simulink model "plant_ode_tmp"  (R2023b)
settings: Solver=VariableStepAuto  StartTime=0.0  StopTime=10.0  RelTol=1e-3
values from neighbouring files (symbols this model uses):
  param = plant_param()    [plot_bode.m]    (also in plot_impulse.m; plot_initial.m)
  x0 = [0;0;50e3;50e3]    [plot_initial.m]
libraries: simulink x4
settings Model: Creator=block  LastModifiedBy=MPC5

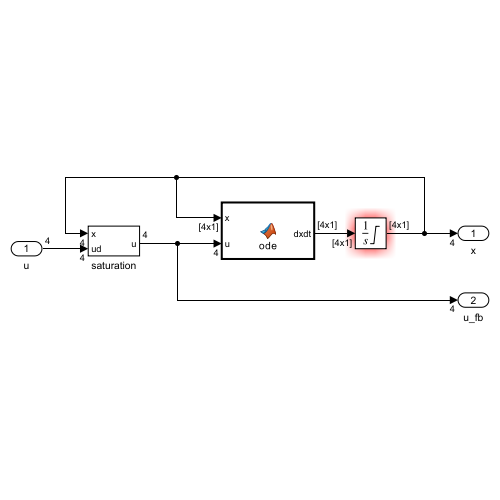
[thumbnail: Simulink's stored preview of the top-level diagram]
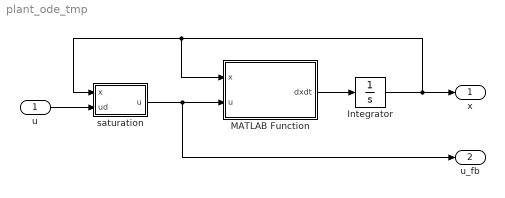
== system plant_ode_tmp ==
  u : Inport  PortDimensions=param.udim
  Integrator : Integrator  InitialCondition=x0  LimitOutput=on  UpperSaturationLimit=[param.L/2;inf;inf;inf]  LowerSaturationLimit=[-param.L/2;-inf;-inf;-inf]
  MATLAB Function : MATLAB Function  TreatAsAtomicUnit=on
  saturation : Subsystem
  x : Outport  PortDimensions=param.xdim
  u_fb : Outport  Port=2  PortDimensions=param.udim
  wires:
  MATLAB Function/1(dxdt) -> Integrator/1
  Integrator/1 -> x/1, MATLAB Function/1(x), saturation/1(x)
  saturation/1(u) -> u_fb/1, MATLAB Function/2(u)
  u/1 -> saturation/2(ud)

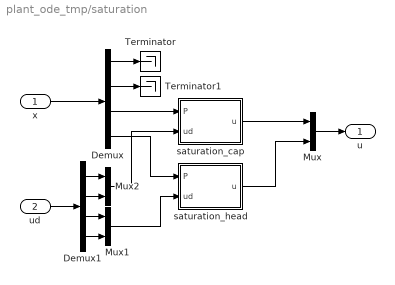
== system plant_ode_tmp/saturation ==
  x : Inport  PortDimensions=param.xdim
  ud : Inport  Port=2  PortDimensions=param.udim
  Demux : Demux
  Demux1 : Demux
  Mux : Mux  Inputs=2
  Mux1 : Mux  Inputs=2
  Mux2 : Mux  Inputs=2
  Terminator : Terminator
  Terminator1 : Terminator
  saturation_cap : Subsystem
  saturation_head : Subsystem
  u : Outport
  wires:
  x/1 -> Demux/1
  Demux/3 -> saturation_cap/1(P)
  Demux/4 -> saturation_head/1(P)
  Demux/1 -> Terminator/1
  Demux/2 -> Terminator1/1
  saturation_cap/1(u) -> Mux/1
  saturation_head/1(u) -> Mux/2
  Mux/1 -> u/1
  ud/1 -> Demux1/1
  Demux1/4 -> Mux1/2
  Demux1/3 -> Mux1/1
  Demux1/1 -> Mux2/1
  Demux1/2 -> Mux2/2
  Mux2/1 -> saturation_cap/2(ud)
  Mux1/1 -> saturation_head/2(ud)

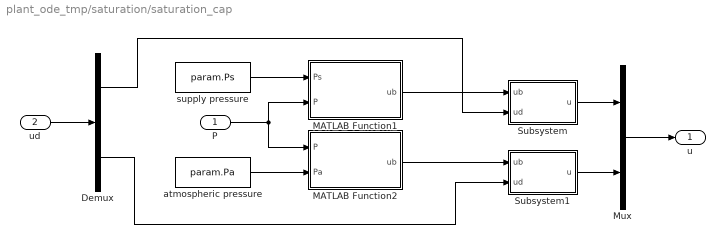
== system plant_ode_tmp/saturation/saturation_cap ==
  P : Inport
  ud : Inport  Port=2
  Demux : Demux  Outputs=2
  MATLAB Function1 : MATLAB Function  TreatAsAtomicUnit=on
  MATLAB Function2 : MATLAB Function  TreatAsAtomicUnit=on
  Mux : Mux  Inputs=2
  Subsystem : Subsystem
  Subsystem1 : Subsystem
  atmospheric pressure : Constant  Value=param.Pa
  supply pressure : Constant  Value=param.Ps
  u : Outport
  wires:
  ud/1 -> Demux/1
  Mux/1 -> u/1
  supply pressure/1 -> MATLAB Function1/1(Ps)
  P/1 -> MATLAB Function1/2(P), MATLAB Function2/1(P)
  atmospheric pressure/1 -> MATLAB Function2/2(Pa)
  MATLAB Function1/1(ub) -> Subsystem/1(ub)
  MATLAB Function2/1(ub) -> Subsystem1/1(ub)
  Demux/1 -> Subsystem/2(ud)
  Demux/2 -> Subsystem1/2(ud)
  Subsystem/1(u) -> Mux/1
  Subsystem1/1(u) -> Mux/2

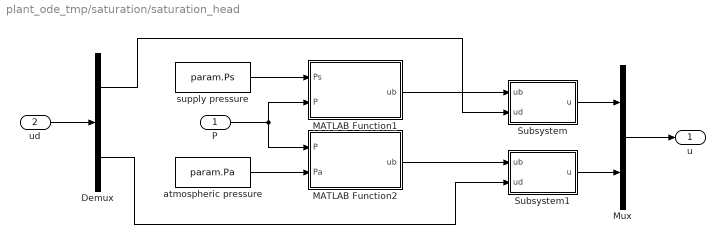
== system plant_ode_tmp/saturation/saturation_head ==
  P : Inport
  ud : Inport  Port=2
  Demux : Demux  Outputs=2
  MATLAB Function1 : MATLAB Function  TreatAsAtomicUnit=on
  MATLAB Function2 : MATLAB Function  TreatAsAtomicUnit=on
  Mux : Mux  Inputs=2
  Subsystem : Subsystem
  Subsystem1 : Subsystem
  atmospheric pressure : Constant  Value=param.Pa
  supply pressure : Constant  Value=param.Ps
  u : Outport
  wires:
  ud/1 -> Demux/1
  Mux/1 -> u/1
  supply pressure/1 -> MATLAB Function1/1(Ps)
  P/1 -> MATLAB Function1/2(P), MATLAB Function2/1(P)
  atmospheric pressure/1 -> MATLAB Function2/2(Pa)
  MATLAB Function1/1(ub) -> Subsystem/1(ub)
  MATLAB Function2/1(ub) -> Subsystem1/1(ub)
  Demux/1 -> Subsystem/2(ud)
  Demux/2 -> Subsystem1/2(ud)
  Subsystem/1(u) -> Mux/1
  Subsystem1/1(u) -> Mux/2

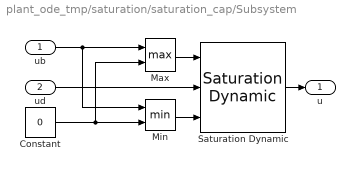
== system plant_ode_tmp/saturation/saturation_cap/Subsystem ==
  ub : Inport
  ud : Inport  Port=2
  Constant : Constant  Value=0
  Max : MinMax  Function=max  Inputs=2
  Min : MinMax  Inputs=2
  Saturation Dynamic : simulink/Discontinuities/Saturation Dynamic  OutMin=[]  OutMax=[]  OutDataTypeStr=Inherit: Same as second input  OutDataType=fixdt(1, 16)  OutScaling=2^-10  DoSatur=off
  u : Outport
  wires:
  Min/1 -> Saturation Dynamic/3
  ud/1 -> Saturation Dynamic/2
  Constant/1 -> Max/2, Min/2
  Max/1 -> Saturation Dynamic/1
  Saturation Dynamic/1 -> u/1
  ub/1 -> Min/1, Max/1

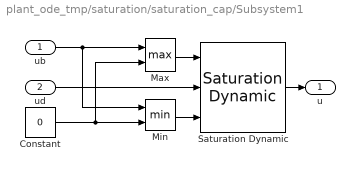
== system plant_ode_tmp/saturation/saturation_cap/Subsystem1 ==
  ub : Inport
  ud : Inport  Port=2
  Constant : Constant  Value=0
  Max : MinMax  Function=max  Inputs=2
  Min : MinMax  Inputs=2
  Saturation Dynamic : simulink/Discontinuities/Saturation Dynamic  OutMin=[]  OutMax=[]  OutDataTypeStr=Inherit: Same as second input  OutDataType=fixdt(1, 16)  OutScaling=2^-10  DoSatur=off
  u : Outport
  wires:
  ub/1 -> Max/1, Min/1
  Saturation Dynamic/1 -> u/1
  Max/1 -> Saturation Dynamic/1
  Constant/1 -> Min/2, Max/2
  ud/1 -> Saturation Dynamic/2
  Min/1 -> Saturation Dynamic/3

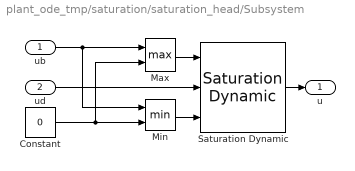
== system plant_ode_tmp/saturation/saturation_head/Subsystem ==
  ub : Inport
  ud : Inport  Port=2
  Constant : Constant  Value=0
  Max : MinMax  Function=max  Inputs=2
  Min : MinMax  Inputs=2
  Saturation Dynamic : simulink/Discontinuities/Saturation Dynamic  OutMin=[]  OutMax=[]  OutDataTypeStr=Inherit: Same as second input  OutDataType=fixdt(1, 16)  OutScaling=2^-10  DoSatur=off
  u : Outport
  wires:
  Min/1 -> Saturation Dynamic/3
  ud/1 -> Saturation Dynamic/2
  Constant/1 -> Max/2, Min/2
  Max/1 -> Saturation Dynamic/1
  Saturation Dynamic/1 -> u/1
  ub/1 -> Min/1, Max/1

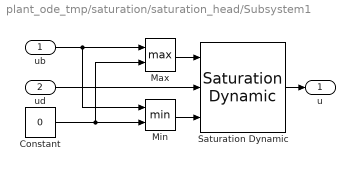
== system plant_ode_tmp/saturation/saturation_head/Subsystem1 ==
  ub : Inport
  ud : Inport  Port=2
  Constant : Constant  Value=0
  Max : MinMax  Function=max  Inputs=2
  Min : MinMax  Inputs=2
  Saturation Dynamic : simulink/Discontinuities/Saturation Dynamic  OutMin=[]  OutMax=[]  OutDataTypeStr=Inherit: Same as second input  OutDataType=fixdt(1, 16)  OutScaling=2^-10  DoSatur=off
  u : Outport
  wires:
  ub/1 -> Max/1, Min/1
  Saturation Dynamic/1 -> u/1
  Max/1 -> Saturation Dynamic/1
  Constant/1 -> Min/2, Max/2
  ud/1 -> Saturation Dynamic/2
  Min/1 -> Saturation Dynamic/3

== matlab function plant_ode_tmp/MATLAB Function ==
  data: x input; u input; dxdt output; param parameter
function dxdt = ode(x,u,param)
    dxdt = plant_ode(0,x,u,param);
end

== matlab function plant_ode_tmp/saturation/saturation_cap/MATLAB Function2 ==
  data: P input; Pa input; ub output; param parameter
function ub = outflow(P,Pa,param)
    ub = input_constraint(P,Pa,param);
end

== matlab function plant_ode_tmp/saturation/saturation_head/MATLAB Function1 ==
  data: Ps input; P input; ub output; param parameter
function ub = inflow(Ps,P,param)
    ub = input_constraint(Ps,P,param);
end

== matlab function plant_ode_tmp/saturation/saturation_head/MATLAB Function2 ==
  data: P input; Pa input; ub output; param parameter
function ub = outflow(P,Pa,param)
    ub = input_constraint(P,Pa,param);
end

== matlab function plant_ode_tmp/saturation/saturation_cap/MATLAB Function1 ==
  data: Ps input; P input; ub output; param parameter
function ub = inflow(Ps,P,param)
    ub = input_constraint(Ps,P,param);
end
